simulink library "PosControl"  (R2024a)
settings: Solver=VariableStepAuto  StartTime=0.0  StopTime=10.0  RelTol=1e-3
undefined symbols (not defined in the file): MOT_THST_HOVER, PSC_ACCZ_D, PSC_ACCZ_D_FF, PSC_ACCZ_FF, PSC_ACCZ_I, PSC_ACCZ_P, PSC_ANGLE_MAX, PSC_Freq, PSC_POSXY_P, PSC_POSZ_P, PSC_VELXY_D, PSC_VELXY_I, PSC_VELXY_P, PSC_VELZ_D, PSC_VELZ_I, PSC_VELZ_P, THR_CLIMB_MAX, THR_SINK_MAX
libraries: ArdupilotFunctions x4, sharedtransform x1
settings Model: Creator=igmso  LastModifiedBy=igmso

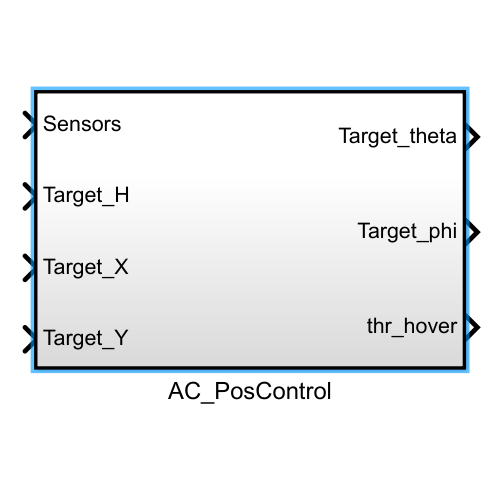
[thumbnail: Simulink's stored preview of the top-level diagram]
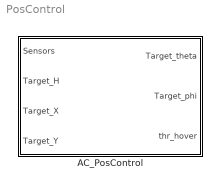
== system PosControl ==
  AC_PosControl : Subsystem  TreatAsAtomicUnit=on

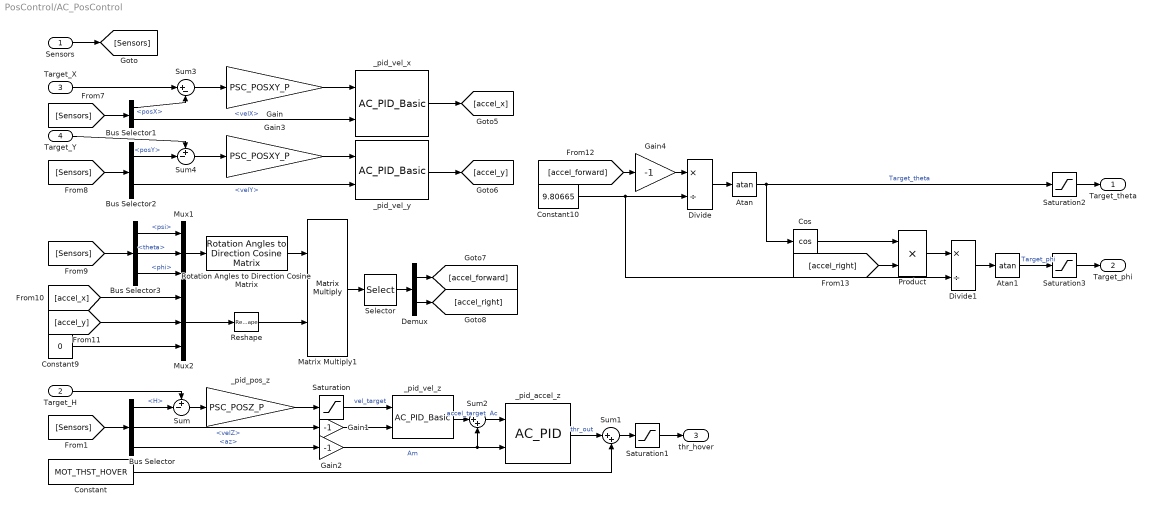
== system PosControl/AC_PosControl ==
  Sensors : Inport  SampleTime=1/PSC_Freq
  Target_H : Inport  Port=2  SampleTime=1/PSC_Freq
  Target_X : Inport  Port=3  SampleTime=1/PSC_Freq
  Target_Y : Inport  Port=4  SampleTime=1/PSC_Freq
  Atan : Trigonometry  Operator=atan
  Atan1 : Trigonometry  Operator=atan
  Bus Selector : BusSelector  OutputSignals=H,velZ,az
  Bus Selector1 : BusSelector  OutputSignals=posX,velX
  Bus Selector2 : BusSelector  OutputSignals=posY,velY
  Bus Selector3 : BusSelector  OutputSignals=psi,theta,phi
  Constant : Constant  Value=MOT_THST_HOVER  SampleTime=-1
  Constant10 : Constant  Value=9.80665  SampleTime=1/PSC_Freq
  Constant9 : Constant  Value=0  SampleTime=1/PSC_Freq
  Cos : Trigonometry  Operator=cos
  Demux : Demux  Outputs=2
  Divide : Product  Inputs=*/
  Divide1 : Product  Inputs=*/
  Gain : Gain  Gain=PSC_POSXY_P
  Gain1 : Gain  Gain=-1
  Gain2 : Gain  Gain=-1
  Gain3 : Gain  Gain=PSC_POSXY_P
  Gain4 : Gain  Gain=-1
  Matrix Multiply1 : Product  Multiplication=Matrix(*)
  Mux1 : Mux  Inputs=3
  Mux2 : Mux  Inputs=3
  Product : Product
  Reshape : Reshape  OutputDimensionality=Column vector (2-D)
  Rotation Angles to Direction Cosine Matrix : sharedtransform/Rotation Angles to Direction Cosine Matrix  rotationOrder=ZYX  aMode=aMode
  Saturation : Saturate  UpperLimit=THR_CLIMB_MAX  LowerLimit=-THR_SINK_MAX
  Saturation1 : Saturate  UpperLimit=1  LowerLimit=0
  Saturation2 : Saturate  UpperLimit=deg2rad(PSC_ANGLE_MAX)  LowerLimit=-deg2rad(PSC_ANGLE_MAX)
  Saturation3 : Saturate
  Selector : Selector  InputPortWidth=3  IndexOptions=Index vector (dialog)  Indices=[1 2]  OutputSizes=1
  Sum : Sum  Inputs=+-|
  Sum1 : Sum  Inputs=|++
  Sum2 : Sum  Inputs=|++
  Sum3 : Sum  Inputs=|+-
  Sum4 : Sum  Inputs=+-|
  _pid_accel_z : ArdupilotFunctions/AC_PID  P=PSC_ACCZ_P  I=PSC_ACCZ_I  D=PSC_ACCZ_D  FF=PSC_ACCZ_FF*1e-3  D_FF=PSC_ACCZ_D_FF*1e-3  FLTD=PSC_ACCZ_FLTD  FLTE=PSC_ACCZ_FLTE  FLTT=PSC_ACCZ_FLTT  IMAX=PSC_ACCZ_IMAX  ControlFreq=PSC_Freq
  _pid_pos_z : Gain  Gain=PSC_POSZ_P
  _pid_vel_x : ArdupilotFunctions/AC_PID_Basic  P=PSC_VELXY_P  I=PSC_VELXY_I  D=PSC_VELXY_D  FF=PSC_VELXY_FF  FLTD=PSC_VELXY_FLTD  FLTE=PSC_VELXY_FLTE  IMAX=PSC_VELXY_IMAX  ControlFreq=PSC_Freq
  _pid_vel_y : ArdupilotFunctions/AC_PID_Basic  P=PSC_VELXY_P  I=PSC_VELXY_I  D=PSC_VELXY_D  FF=PSC_VELXY_FF  FLTD=PSC_VELXY_FLTD  FLTE=PSC_VELXY_FLTE  IMAX=PSC_VELXY_IMAX  ControlFreq=PSC_Freq
  _pid_vel_z : ArdupilotFunctions/AC_PID_Basic  P=PSC_VELZ_P  I=PSC_VELZ_I  D=PSC_VELZ_D  FF=PSC_VELZ_FF  FLTD=PSC_VELZ_FLTD  FLTE=PSC_VELZ_FLTE  IMAX=PSC_VELZ_IMAX  ControlFreq=PSC_Freq
  Target_theta : Outport
  Target_phi : Outport  Port=2
  thr_hover : Outport  Port=3  SampleTime=1/PSC_Freq
  wires:
  Target_H/1 -> Sum/1
  Target_Y/1 -> Sum4/1
  Target_X/1 -> Sum3/1
  _pid_vel_x/1 -> [accel_x]
  Sum3/1 -> Gain/1
  Saturation3/1 -> Target_phi/1
  Saturation2/1 -> Target_theta/1
  Gain/1 -> _pid_vel_x/1
  Sensors/1 -> [Sensors]
  Matrix Multiply1/1 -> Selector/1
  [Sensors] -> Bus Selector2/1
  Gain3/1 -> _pid_vel_y/1
  Bus Selector3/3 -> Mux1/3  "<phi>"
  Bus Selector3/2 -> Mux1/2  "<theta>"
  [accel_x] -> Mux2/1
  Atan/1 -> Cos/1, Saturation2/1  "Target_theta"
  Bus Selector1/2 -> _pid_vel_x/2  "<velX>"
  Constant10/1 -> Divide/2, Divide1/2
  Mux2/1 -> Reshape/1
  [accel_right] -> Product/2
  Atan1/1 -> Saturation3/1  "Target_phi"
  Demux/2 -> [accel_right]
  _pid_vel_y/1 -> [accel_y]
  Bus Selector2/2 -> _pid_vel_y/2  "<velY>"
  Bus Selector2/1 -> Sum4/2  "<posY>"
  [Sensors] -> Bus Selector1/1
  Gain4/1 -> Divide/1
  [accel_forward] -> Gain4/1
  Rotation Angles to Direction Cosine Matrix/1 -> Matrix Multiply1/1
  Selector/1 -> Demux/1
  Bus Selector1/1 -> Sum3/2  "<posX>"
  Cos/1 -> Product/1
  Divide1/1 -> Atan1/1
  [accel_y] -> Mux2/2
  Demux/1 -> [accel_forward]
  Constant9/1 -> Mux2/3
  [Sensors] -> Bus Selector3/1
  Reshape/1 -> Matrix Multiply1/2
  Product/1 -> Divide1/1
  Sum4/1 -> Gain3/1
  Divide/1 -> Atan/1
  Mux1/1 -> Rotation Angles to Direction Cosine Matrix/1
  Bus Selector3/1 -> Mux1/1  "<psi>"
  Saturation/1 -> _pid_vel_z/1  "vel_target"
  Sum2/1 -> _pid_accel_z/1  "Ac"
  _pid_vel_z/1 -> Sum2/1  "accel_target"
  Gain2/1 -> _pid_accel_z/2, Sum2/2  "Am"
  Constant/1 -> Sum1/2
  _pid_accel_z/1 -> Sum1/1  "thr_out"
  Bus Selector/3 -> Gain2/1  "<az>"
  Bus Selector/2 -> Gain1/1  "<velZ>"
  _pid_pos_z/1 -> Saturation/1
  Sum/1 -> _pid_pos_z/1
  Bus Selector/1 -> Sum/2  "<H>"
  [Sensors] -> Bus Selector/1
  Sum1/1 -> Saturation1/1
  Gain1/1 -> _pid_vel_z/2
  Saturation1/1 -> thr_hover/1
